simulink model "question3"  (R2019b)
settings: Solver=VariableStepAuto  StartTime=0.0  StopTime=1  RelTol=1e-3
settings Model: Creator=theojanson  LastModifiedBy=theojanson

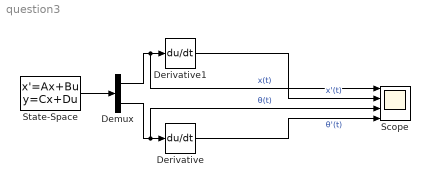
== system question3 ==
  Demux : Demux  Outputs=2
  Derivative : Derivative
  Derivative1 : Derivative
  Scope : Scope  NumInputPorts=4
  State-Space : StateSpace  A=[0 1 0 0 ; 0 -14.4899 -1.9749 0 ; 0 0 0 1 ; 0 86.2495 58.3333 0]  B=[0 ; 3.255 ; 0 ; -19.3751]  C=[1 0 0 0 ; 0 0 1 0]  D=[0;0]  InitialCondition=[0,0,0.05,0]
  wires:
  State-Space/1 -> Demux/1
  Demux/1 -> Scope/1, Derivative1/1  "x(t)"
  Demux/2 -> Scope/3, Derivative/1  "θ(t)"
  Derivative1/1 -> Scope/2  "x'(t)"
  Derivative/1 -> Scope/4  "θ'(t)"
